simulink model "MI6FS_HE_6PhS"  (R2023a)
settings: Solver=FixedStepAuto  StartTime=0  StopTime=L  FixedStep=Ts  RelTol=1e-3
values from neighbouring files (symbols this model uses):
  A = exp(j*pi/3)    [Parameters.m]
  deg = 0    [Parameters.m]
  FV = 9.8    [Parameters.m]
  J = 0.0243    [Parameters.m]
  Lrr = [((1/3*Lm)+Llr) 1/6*Lm -1/6*Lm -1/3*Lm -1/6*Lm 1/6*Lm;        1/6*Lm ((1/3*Lm)+Llr) 1/6*Lm -1/6*Lm -1/3*Lm -1/6*Lm;        -1/6*Lm 1/6*Lm ((1/3*Lm)+Llr) 1/6*Lm -1/6*Lm -1/3*Lm;        -1/3*Lm -1/6*Lm 1/6*Lm ((1/3*Lm)+Llr) 1/6*Lm -1/6*Lm;        -1/6*Lm -1/3*Lm -1/6*Lm 1/6*Lm ((1/3*Lm)+Llr) 1/6*Lm;        1/6*Lm -1/6*Lm -1/3*Lm -1/6*Lm 1/6*Lm ((1/3*Lm)+Llr)]    [Parameters.m]
  Lrs = transpose(Lsr)    [Parameters.m]
  Lsr = [0 (pi/3) 2*(pi/3) 3*(pi/3) 4*(pi/3) 5*(pi/3);        -(pi/3) 0 (pi/3) 2*(pi/3) 3*(pi/3) 4*(pi/3);        -2*(pi/3) -(pi/3) 0 (pi/3) 2*(pi/3) 3*(pi/3);        -3*(pi/3) -2*(pi/3) -(pi/3) 0 (pi/3) 2*(pi/3);        -4*(pi/3) -3*(pi/3) -2*(pi/3) -(pi/3) 0 (pi/3);        -5*(pi/3) -4*(pi/3) -3*(pi/3) -2*(pi/3) -(pi/3) 0]    [Parameters.m]
  Lss = [((1/3*Lm)+Lls) 1/6*Lm -1/6*Lm -1/3*Lm -1/6*Lm 1/6*Lm;        1/6*Lm ((1/3*Lm)+Lls) 1/6*Lm -1/6*Lm -1/3*Lm -1/6*Lm;        -1/6*Lm 1/6*Lm ((1/3*Lm)+Lls) 1/6*Lm -1/6*Lm -1/3*Lm;        -1/3*Lm -1/6*Lm 1/6*Lm ((1/3*Lm)+Lls) 1/6*Lm -1/6*Lm;        -1/6*Lm -1/3*Lm -1/6*Lm 1/6*Lm ((1/3*Lm)+Lls) 1/6*Lm;        1/6*Lm -1/6*Lm -1/3*Lm -1/6*Lm 1/6*Lm ((1/3*Lm)+Lls)]    [Parameters.m]
  Lto = 0    [Parameters.m]
  Msr = (1/3)*Lm    (= 0.0620333333333)    [Parameters.m]
  p = 2    [Parameters.m]
  Rcore = 811    [Parameters.m]
  Rrr = Rr*eye(6,6)    [Parameters.m]
  Rss = Rs*eye(6,6)    [Parameters.m]
  Tav = 0.23    [Parameters.m]
  Ts = 1/Fs    (= 1e-05)    [Parameters.m]
  Us = sqrt(2)*180    [Parameters.m]
undefined symbols (not defined in the file or in its folder): DiscIntNeverNeededParam, j
libraries: spsFourierLib x84, spsVoltageMeasurementLib x13, spsACVoltageSourceLib x6, spsControlledCurrentSourceLib x6, spsCurrentMeasurementLib x6, spsSeriesRLCBranchLib x6, spsSequenceAnalyzerLib x6, sharedutil x5, eeRmsMeasurement x2, eeGeneralControl x1, spsSequenceAnalyzerPhasorLib x1, spsabctoAlphaBetaZeroLib x1
(part 3 of 3)

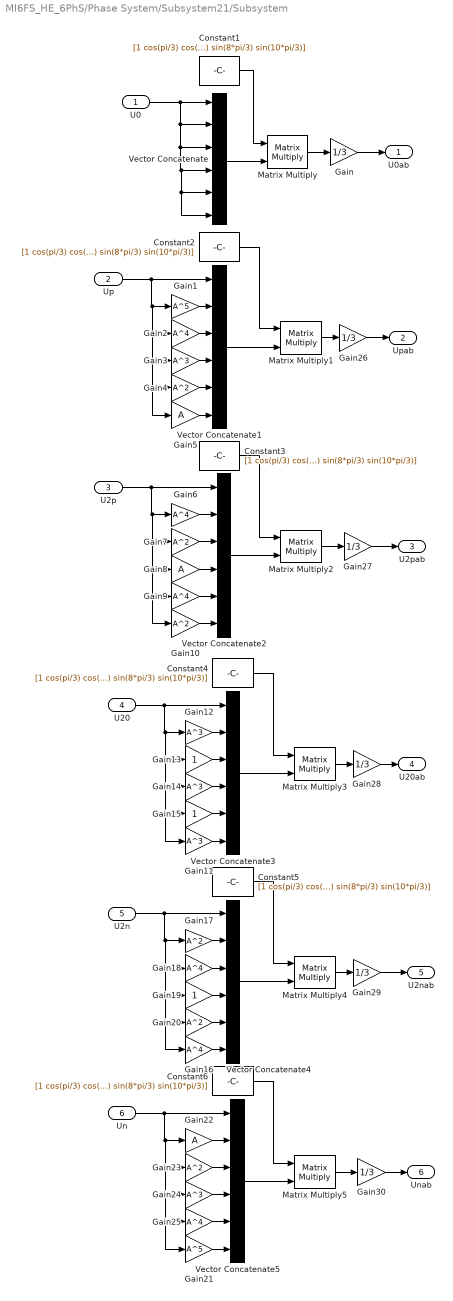
== system MI6FS_HE_6PhS/Phase System/Subsystem21/Subsystem ==
  U0 : Inport
  Up : Inport  Port=2
  U2p : Inport  Port=3
  U20 : Inport  Port=4
  U2n : Inport  Port=5
  Un : Inport  Port=6
  Constant{1..6} (6 alike) : Constant  Value=[1 cos(pi/3) cos(2*pi/3) cos(3*pi/3) cos(4*pi/3) cos(5*pi/3); 0 sin(pi/3) sin(2*pi/3) sin(3*pi/3) sin(4*pi/3) sin(5*pi/3); 1 cos(2*pi/3) cos(4*pi/3) cos(6*pi/3) cos(8*pi/3) cos(10*pi/3);1 sin(2*pi/3) sin(4*pi/3) sin(6*pi/3) sin(8*pi/3) sin(10*pi/3)]
  Gain{,26..30} (6 alike) : Gain  Gain=1/3
  Gain1 : Gain  Gain=A^5
  Gain{4,7,10,17,20,23} (6 alike) : Gain  Gain=A^2
  Gain{3,11..12,14,24} (5 alike) : Gain  Gain=A^3
  Gain13 : Gain
  Gain15 : Gain
  Gain{2,6,9,16,18,25} (6 alike) : Gain  Gain=A^4
  Gain19 : Gain
  Gain21 : Gain  Gain=A^5
  Gain22 : Gain  Gain=A
  Gain5 : Gain  Gain=A
  Gain8 : Gain  Gain=A
  Matrix Multiply{,1..5} (6 alike) : Product  Multiplication=Matrix(*)
  Vector Concatenate{,1..5} (6 alike) : Concatenate  NumInputs=6
  U0ab : Outport
  Upab : Outport  Port=2
  U2pab : Outport  Port=3
  U20ab : Outport  Port=4
  U2nab : Outport  Port=5
  Unab : Outport  Port=6
  wires:
  Gain30/1 -> Unab/1
  Matrix Multiply5/1 -> Gain30/1
  Gain29/1 -> U2nab/1
  Matrix Multiply4/1 -> Gain29/1
  Matrix Multiply3/1 -> Gain28/1
  Gain28/1 -> U20ab/1
  Gain27/1 -> U2pab/1
  Matrix Multiply2/1 -> Gain27/1
  Matrix Multiply1/1 -> Gain26/1
  Gain26/1 -> Upab/1
  Gain/1 -> U0ab/1
  Gain22/1 -> Vector Concatenate5/2
  Gain25/1 -> Vector Concatenate5/5
  Constant6/1 -> Matrix Multiply5/1
  Un/1 -> Gain22/1, Gain23/1, Gain24/1, Gain25/1, Gain21/1, Vector Concatenate5/1
  Gain21/1 -> Vector Concatenate5/6
  Gain24/1 -> Vector Concatenate5/4
  Vector Concatenate5/1 -> Matrix Multiply5/2
  Gain23/1 -> Vector Concatenate5/3
  Gain18/1 -> Vector Concatenate4/3
  Gain19/1 -> Vector Concatenate4/4
  Vector Concatenate4/1 -> Matrix Multiply4/2
  U2n/1 -> Gain17/1, Gain18/1, Gain19/1, Gain20/1, Gain16/1, Vector Concatenate4/1
  Gain20/1 -> Vector Concatenate4/5
  Constant5/1 -> Matrix Multiply4/1
  Gain16/1 -> Vector Concatenate4/6
  Gain17/1 -> Vector Concatenate4/2
  Gain11/1 -> Vector Concatenate3/6
  Gain14/1 -> Vector Concatenate3/4
  Constant4/1 -> Matrix Multiply3/1
  Gain12/1 -> Vector Concatenate3/2
  Gain15/1 -> Vector Concatenate3/5
  U20/1 -> Gain12/1, Gain13/1, Gain14/1, Gain15/1, Gain11/1, Vector Concatenate3/1
  Vector Concatenate3/1 -> Matrix Multiply3/2
  Gain13/1 -> Vector Concatenate3/3
  Vector Concatenate2/1 -> Matrix Multiply2/2
  Gain7/1 -> Vector Concatenate2/3
  U2p/1 -> Gain6/1, Gain7/1, Gain8/1, Gain9/1, Gain10/1, Vector Concatenate2/1
  Constant3/1 -> Matrix Multiply2/1
  Gain10/1 -> Vector Concatenate2/6
  Gain9/1 -> Vector Concatenate2/5
  Gain6/1 -> Vector Concatenate2/2
  Gain8/1 -> Vector Concatenate2/4
  Constant2/1 -> Matrix Multiply1/1
  Vector Concatenate1/1 -> Matrix Multiply1/2
  Gain5/1 -> Vector Concatenate1/6
  Gain4/1 -> Vector Concatenate1/5
  Gain3/1 -> Vector Concatenate1/4
  Gain2/1 -> Vector Concatenate1/3
  Gain1/1 -> Vector Concatenate1/2
  Up/1 -> Vector Concatenate1/1, Gain1/1, Gain2/1, Gain3/1, Gain4/1, Gain5/1
  Matrix Multiply/1 -> Gain/1
  Constant1/1 -> Matrix Multiply/1
  Vector Concatenate/1 -> Matrix Multiply/2
  U0/1 -> Vector Concatenate/5, Vector Concatenate/6, Vector Concatenate/4, Vector Concatenate/3, Vector Concatenate/2, Vector Concatenate/1

== system MI6FS_HE_6PhS/Phase System/Subsystem3/-wt ==
  Bias2 : Bias  Bias=-2*pi*2*50*Ts  SaturateOnIntegerOverflow=off
  Scope22 : Scope
  Unit Delay : UnitDelay  SampleTime=-1  HasFrameUpgradeWarning=on
  -wt : Outport
  wires:
  Bias2/1 -> Unit Delay/1, Scope22/1, -wt/1
  Unit Delay/1 -> Bias2/1

== system MI6FS_HE_6PhS/Phase System/Subsystem5/-wt ==
  Bias2 : Bias  Bias=2*pi*50*Ts  SaturateOnIntegerOverflow=off
  Scope22 : Scope
  Unit Delay : UnitDelay  SampleTime=-1  HasFrameUpgradeWarning=on
  -wt : Outport
  wires:
  Bias2/1 -> Unit Delay/1, Scope22/1, -wt/1
  Unit Delay/1 -> Bias2/1
